simulink model "two_states_with_two_substates"  (R2017b)
settings: Solver=FixedStepDiscrete  StartTime=0.0  StopTime=10.0  RelTol=1e-3
settings Model: Creator=flosch  LastModifiedBy=flosch
settings ConfigComp: CovScope=ReferencedModels  CovIncludeTopModel=off

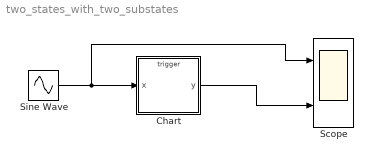
== system two_states_with_two_substates ==
  Chart : Stateflow chart  TreatAsAtomicUnit=on
  Scope : Scope  NumInputPorts=2
  Sine Wave : Sin  SampleTime=0
  wires:
  Sine Wave/1 -> Scope/1, Chart/1(x)
  Chart/1(y) -> Scope/2

== stateflow chart two_states_with_two_substates/Chart ==
  state Big_Kitten
    state Kitten
      entry: y = 0;
    state Potato
      entry: y = 1;
    (default) -> Kitten
    Kitten -> Potato : Event_B
  state Big_Potato
    state Fish
      entry: y = 2;
    state Horse
      entry: y = x;
    state Lemon
      entry: y = -x;
    (default) -> Fish
    Fish -> Horse [order 1] : Event_B [x > 0]
    Fish -> Lemon [order 2] : Event_B [x < 0]
  note: cyc = 15
  (default) -> Big_Kitten
  Big_Kitten -> Big_Potato : Event_A
  Big_Potato -> Big_Kitten : Event_A
  data: t0 constant double =0.0; x input; y output
  events: Event_A input FUNCTION_CALL_EVENT; Event_B input FUNCTION_CALL_EVENT
